simulink model "VelocityTransitionHandler"  (R2016b)
settings: Solver=FixedStepAuto  StartTime=0.0  StopTime=10.0  FixedStep=0.002  RelTol=1e-3  EnableMultiTasking=on
libraries: simulink x1
settings Model: Creator=march  LastModifiedBy=march
settings SolverCC: EnableConcurrentExecution=on
settings DataIOCC: SaveFormat=StructureWithTime
settings OptimizationCC: BlockReduction=off  OptimizeBlockIOStorage=off  BufferReuse=off  GlobalBufferReuse=off  ExpressionFolding=off  LocalBlockOutputs=off
settings HardwareCC: ProdBitPerPointer=32  ProdBitPerSizeT=32  ProdBitPerPtrDiffT=32  ProdLargestAtomicFloat=None  ProdWordSize=32  ProdLongLongMode=on  ProdHWDeviceType=Generic->32-bit x86 compatible
settings RTWCC: SystemTargetFile=slrt.tlc  TemplateMakefile=slrt_default_tmf  Description=Simulink Real-Time  RTWCompilerOptimization=on

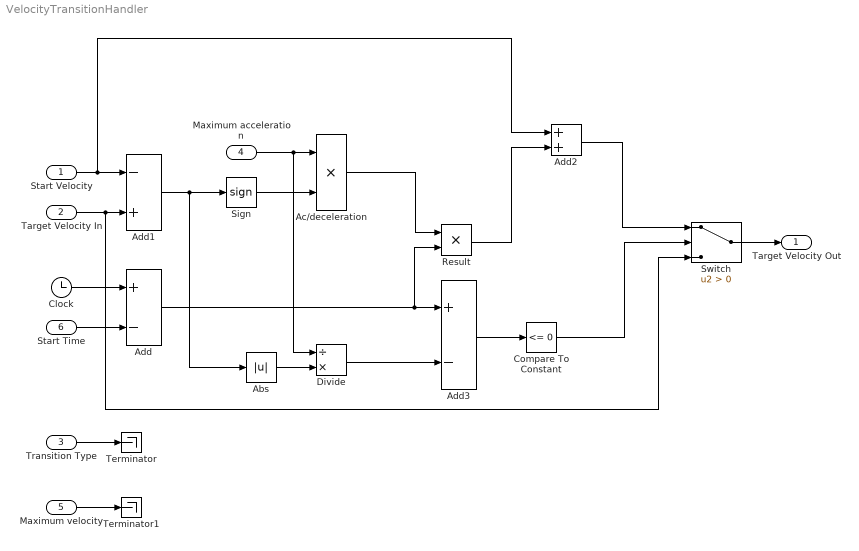
== system VelocityTransitionHandler ==
  Start Velocity : Inport
  Target Velocity In : Inport  Port=2
  Transition Type : Inport  Port=3
  Maximum acceleration : Inport  Port=4
  Maximum velocity : Inport  Port=5
  Start Time : Inport  Port=6
  Abs : Abs
  Ac/deceleration : Product  Inputs=**
  Add : Sum  Inputs=+-
  Add1 : Sum  Inputs=-+
  Add2 : Sum
  Add3 : Sum  Inputs=+-
  Clock : Clock
  Compare To Constant : simulink/Logic and Bit Operations/Compare To Constant  relop=<=  const=0  OutDataTypeStr=boolean
  Divide : Product  Inputs=/*
  Result : Product  Inputs=**
  Sign : Signum
  Switch : Switch  Criteria=u2 > Threshold
  Terminator : Terminator
  Terminator1 : Terminator
  Target Velocity Out : Outport
  wires:
  Clock/1 -> Add/1
  Start Time/1 -> Add/2
  Start Velocity/1 -> Add2/1, Add1/1
  Target Velocity In/1 -> Switch/3, Add1/2
  Add1/1 -> Abs/1, Sign/1
  Ac/deceleration/1 -> Result/1
  Add/1 -> Add3/1, Result/2
  Sign/1 -> Ac/deceleration/2
  Maximum acceleration/1 -> Divide/1, Ac/deceleration/1
  Maximum velocity/1 -> Terminator1/1
  Transition Type/1 -> Terminator/1
  Result/1 -> Add2/2
  Add2/1 -> Switch/1
  Abs/1 -> Divide/2
  Divide/1 -> Add3/2
  Add3/1 -> Compare To Constant/1
  Compare To Constant/1 -> Switch/2
  Switch/1 -> Target Velocity Out/1
